simulink model "Parallel_n64"  (R2012b)
settings: Solver=VariableStepDiscrete  StartTime=0.0  StopTime=TotalIterations  RelTol=1e-3
values from neighbouring files (symbols this model uses):
  bp = 12    [ConfigValidate.m]
  bpSNMemory = bp    (= 12)    [ConfigValidate.m]
  IterationsOrdering = 4000    [ConfigValidate.m]
  MaxCoordDistance = (abs(max(wx) - min(wx))+abs(max(wy) - min(wy)))^2    [ConfigValidate.m]
  N_limit = 0.01    [ConfigValidate.m]
  nBits = 9    [ConfigValidate.m]
  nBitsNSmemories = (ceil(log2(TotalIterations)))    [ConfigValidate.m]
  S_limit = 1    [ConfigValidate.m]
  SourceNodes = 2000    [ConfigValidate.m]
  ts = 1    [ConfigValidate.m]
  w1 = rand(1,Neurons)    [ConfigValidate.m]
  w2 = rand(1,Neurons)    [ConfigValidate.m]
  wx = zeros(1,Neurons)    [ConfigValidate.m]
  wy = zeros(1,Neurons)    [ConfigValidate.m]
  x1 = rand(SourceNodes,1)    [ConfigValidate.m]
  x2 = rand(SourceNodes,1)    [ConfigValidate.m]
libraries: xbsIndex_r4 x6367, dspsrcs4 x2, dspstat3 x2
(part 19 of 28)

== system Parallel_n64/WiningNeuronFinder1/LowerDist_n17 ==
  In1 : Inport
  In2 : Inport  Port=2
  In3 : Inport  Port=3
  In4 : Inport  Port=4
  In5 : Inport  Port=5
  In6 : Inport  Port=6
  In7 : Inport  Port=7
  In8 : Inport  Port=8
  In9 : Inport  Port=9
  In10 : Inport  Port=10
  In11 : Inport  Port=11
  In12 : Inport  Port=12
  In13 : Inport  Port=13
  In14 : Inport  Port=14
  In15 : Inport  Port=15
  In16 : Inport  Port=16
  In17 : Inport  Port=17
  In18 : Inport  Port=18
  In19 : Inport  Port=19
  In20 : Inport  Port=20
  In21 : Inport  Port=21
  In22 : Inport  Port=22
  In23 : Inport  Port=23
  In24 : Inport  Port=24
  In25 : Inport  Port=25
  In26 : Inport  Port=26
  In27 : Inport  Port=27
  In28 : Inport  Port=28
  In29 : Inport  Port=29
  In30 : Inport  Port=30
  In31 : Inport  Port=31
  In32 : Inport  Port=32
  In33 : Inport  Port=33
  In34 : Inport  Port=34
  In35 : Inport  Port=35
  In36 : Inport  Port=36
  In37 : Inport  Port=37
  In38 : Inport  Port=38
  In39 : Inport  Port=39
  In40 : Inport  Port=40
  In41 : Inport  Port=41
  In42 : Inport  Port=42
  In43 : Inport  Port=43
  In44 : Inport  Port=44
  In45 : Inport  Port=45
  In46 : Inport  Port=46
  In47 : Inport  Port=47
  In48 : Inport  Port=48
  In49 : Inport  Port=49
  In50 : Inport  Port=50
  In51 : Inport  Port=51
  In52 : Inport  Port=52
  In53 : Inport  Port=53
  In54 : Inport  Port=54
  In55 : Inport  Port=55
  In56 : Inport  Port=56
  In57 : Inport  Port=57
  In58 : Inport  Port=58
  In59 : Inport  Port=59
  In60 : Inport  Port=60
  In61 : Inport  Port=61
  In62 : Inport  Port=62
  In63 : Inport  Port=63
  In64 : Inport  Port=64
  Dist_compare{,1..62} (63 alike) : xbsIndex_r4/Relational  mode=a<=b  en=off  latency=dComparator_CompetitiveProcess  dbl_ovrd=off  block_type=relational
  Logical : xbsIndex_r4/Logical  logical_function=AND  inputs=63  en=off  latency=0  precision=Full  arith_type=Unsigned  n_bits=16  bin_pt=0  align_bp=on  dbl_ovrd=off  block_type=logical
  Out1 : Outport
  wires:
  In24/1 -> Dist_compare19/2
  In23/1 -> Dist_compare18/2
  In17/1 -> Dist_compare15/2
  In16/1 -> Dist_compare14/2
  In14/1 -> Dist_compare12/2
  In12/1 -> Dist_compare10/2
  In11/1 -> Dist_compare9/2
  In10/1 -> Dist_compare8/2
  In8/1 -> Dist_compare6/2
  In22/1 -> Dist_compare17/2
  In13/1 -> Dist_compare11/2
  In9/1 -> Dist_compare7/2
  In20/1 -> Dist_compare24/2
  In21/1 -> Dist_compare16/2
  In19/1 -> Dist_compare23/2
  In18/1 -> Dist_compare22/2
  In25/1 -> Dist_compare20/2
  In15/1 -> Dist_compare13/2
  In2/1 -> Dist_compare/2
  In7/1 -> Dist_compare5/2
  In5/1 -> Dist_compare2/2
  In6/1 -> Dist_compare3/2
  In4/1 -> Dist_compare4/2
  In3/1 -> Dist_compare1/2
  Dist_compare6/1 -> Logical/7
  Dist_compare16/1 -> Logical/20
  Dist_compare14/1 -> Logical/15
  Dist_compare1/1 -> Logical/2
  Dist_compare11/1 -> Logical/12
  Dist_compare/1 -> Logical/1
  Dist_compare24/1 -> Logical/19
  Dist_compare13/1 -> Logical/14
  Dist_compare7/1 -> Logical/8
  Dist_compare4/1 -> Logical/5
  Dist_compare9/1 -> Logical/10
  Dist_compare5/1 -> Logical/6
  Dist_compare18/1 -> Logical/22
  Dist_compare10/1 -> Logical/11
  Dist_compare15/1 -> Logical/16
  Dist_compare23/1 -> Logical/18
  Dist_compare17/1 -> Logical/21
  Dist_compare12/1 -> Logical/13
  Dist_compare20/1 -> Logical/24
  Dist_compare19/1 -> Logical/23
  Logical/1 -> Out1/1
  Dist_compare2/1 -> Logical/3
  Dist_compare22/1 -> Logical/17
  Dist_compare8/1 -> Logical/9
  Dist_compare3/1 -> Logical/4
  In48/1 -> Dist_compare35/2
  In47/1 -> Dist_compare34/2
  In41/1 -> Dist_compare31/2
  In40/1 -> Dist_compare30/2
  In38/1 -> Dist_compare28/2
  In36/1 -> Dist_compare26/2
  In35/1 -> Dist_compare47/2
  In34/1 -> Dist_compare46/2
  In32/1 -> Dist_compare44/2
  In46/1 -> Dist_compare33/2
  In37/1 -> Dist_compare27/2
  In33/1 -> Dist_compare45/2
  In44/1 -> Dist_compare40/2
  In45/1 -> Dist_compare32/2
  In43/1 -> Dist_compare39/2
  In42/1 -> Dist_compare38/2
  In49/1 -> Dist_compare37/2
  In39/1 -> Dist_compare29/2
  In26/1 -> Dist_compare21/2
  In31/1 -> Dist_compare43/2
  In28/1 -> Dist_compare36/2
  In29/1 -> Dist_compare41/2
  In30/1 -> Dist_compare42/2
  In27/1 -> Dist_compare25/2
  In63/1 -> Dist_compare57/2
  In62/1 -> Dist_compare56/2
  In56/1 -> Dist_compare53/2
  In55/1 -> Dist_compare52/2
  In53/1 -> Dist_compare50/2
  In51/1 -> Dist_compare48/2
  In50/1 -> Dist_compare62/2
  In61/1 -> Dist_compare55/2
  In52/1 -> Dist_compare49/2
  In59/1 -> Dist_compare61/2
  In60/1 -> Dist_compare54/2
  In58/1 -> Dist_compare60/2
  In57/1 -> Dist_compare59/2
  In64/1 -> Dist_compare58/2
  In54/1 -> Dist_compare51/2
  In1/1 -> Dist_compare58/1, Dist_compare57/1, Dist_compare56/1, Dist_compare55/1, Dist_compare54/1, Dist_compare61/1, Dist_compare60/1, Dist_compare59/1, Dist_compare53/1, Dist_compare52/1, Dist_compare51/1, Dist_compare50/1, Dist_compare49/1, Dist_compare48/1, Dist_compare62/1, Dist_compare37/1, Dist_compare35/1, Dist_compare34/1, Dist_compare33/1, Dist_compare32/1, Dist_compare40/1, Dist_compare39/1, Dist_compare38/1, Dist_compare31/1, Dist_compare30/1, Dist_compare29/1, Dist_compare28/1, Dist_compare27/1, Dist_compare26/1, Dist_compare47/1, Dist_compare46/1, Dist_compare45/1, Dist_compare44/1, Dist_compare43/1, Dist_compare42/1, Dist_compare41/1, Dist_compare36/1, Dist_compare25/1, Dist_compare21/1, Dist_compare20/1, Dist_compare19/1, Dist_compare18/1, Dist_compare17/1, Dist_compare16/1, Dist_compare24/1, Dist_compare23/1, Dist_compare22/1, Dist_compare15/1, Dist_compare14/1, Dist_compare13/1, Dist_compare12/1, Dist_compare11/1, Dist_compare10/1, Dist_compare9/1, Dist_compare8/1, Dist_compare7/1, Dist_compare6/1, Dist_compare5/1, Dist_compare4/1, Dist_compare3/1, Dist_compare2/1, Dist_compare1/1, Dist_compare/1
  Dist_compare21/1 -> Logical/25
  Dist_compare25/1 -> Logical/26
  Dist_compare36/1 -> Logical/27
  Dist_compare41/1 -> Logical/28
  Dist_compare42/1 -> Logical/29
  Dist_compare43/1 -> Logical/30
  Dist_compare44/1 -> Logical/31
  Dist_compare45/1 -> Logical/32
  Dist_compare46/1 -> Logical/33
  Dist_compare47/1 -> Logical/34
  Dist_compare26/1 -> Logical/35
  Dist_compare27/1 -> Logical/36
  Dist_compare28/1 -> Logical/37
  Dist_compare29/1 -> Logical/38
  Dist_compare30/1 -> Logical/39
  Dist_compare31/1 -> Logical/40
  Dist_compare38/1 -> Logical/41
  Dist_compare39/1 -> Logical/42
  Dist_compare40/1 -> Logical/43
  Dist_compare32/1 -> Logical/44
  Dist_compare33/1 -> Logical/45
  Dist_compare34/1 -> Logical/46
  Dist_compare62/1 -> Logical/49
  Dist_compare35/1 -> Logical/47
  Dist_compare48/1 -> Logical/50
  Dist_compare37/1 -> Logical/48
  Dist_compare50/1 -> Logical/52
  Dist_compare49/1 -> Logical/51
  Dist_compare51/1 -> Logical/53
  Dist_compare52/1 -> Logical/54
  Dist_compare53/1 -> Logical/55
  Dist_compare59/1 -> Logical/56
  Dist_compare60/1 -> Logical/57
  Dist_compare61/1 -> Logical/58
  Dist_compare54/1 -> Logical/59
  Dist_compare56/1 -> Logical/61
  Dist_compare55/1 -> Logical/60
  Dist_compare57/1 -> Logical/62
  Dist_compare58/1 -> Logical/63

== system Parallel_n64/WiningNeuronFinder1/LowerDist_n18 ==
  In1 : Inport
  In2 : Inport  Port=2
  In3 : Inport  Port=3
  In4 : Inport  Port=4
  In5 : Inport  Port=5
  In6 : Inport  Port=6
  In7 : Inport  Port=7
  In8 : Inport  Port=8
  In9 : Inport  Port=9
  In10 : Inport  Port=10
  In11 : Inport  Port=11
  In12 : Inport  Port=12
  In13 : Inport  Port=13
  In14 : Inport  Port=14
  In15 : Inport  Port=15
  In16 : Inport  Port=16
  In17 : Inport  Port=17
  In18 : Inport  Port=18
  In19 : Inport  Port=19
  In20 : Inport  Port=20
  In21 : Inport  Port=21
  In22 : Inport  Port=22
  In23 : Inport  Port=23
  In24 : Inport  Port=24
  In25 : Inport  Port=25
  In26 : Inport  Port=26
  In27 : Inport  Port=27
  In28 : Inport  Port=28
  In29 : Inport  Port=29
  In30 : Inport  Port=30
  In31 : Inport  Port=31
  In32 : Inport  Port=32
  In33 : Inport  Port=33
  In34 : Inport  Port=34
  In35 : Inport  Port=35
  In36 : Inport  Port=36
  In37 : Inport  Port=37
  In38 : Inport  Port=38
  In39 : Inport  Port=39
  In40 : Inport  Port=40
  In41 : Inport  Port=41
  In42 : Inport  Port=42
  In43 : Inport  Port=43
  In44 : Inport  Port=44
  In45 : Inport  Port=45
  In46 : Inport  Port=46
  In47 : Inport  Port=47
  In48 : Inport  Port=48
  In49 : Inport  Port=49
  In50 : Inport  Port=50
  In51 : Inport  Port=51
  In52 : Inport  Port=52
  In53 : Inport  Port=53
  In54 : Inport  Port=54
  In55 : Inport  Port=55
  In56 : Inport  Port=56
  In57 : Inport  Port=57
  In58 : Inport  Port=58
  In59 : Inport  Port=59
  In60 : Inport  Port=60
  In61 : Inport  Port=61
  In62 : Inport  Port=62
  In63 : Inport  Port=63
  In64 : Inport  Port=64
  Dist_compare{,1..62} (63 alike) : xbsIndex_r4/Relational  mode=a<=b  en=off  latency=dComparator_CompetitiveProcess  dbl_ovrd=off  block_type=relational
  Logical : xbsIndex_r4/Logical  logical_function=AND  inputs=63  en=off  latency=0  precision=Full  arith_type=Unsigned  n_bits=16  bin_pt=0  align_bp=on  dbl_ovrd=off  block_type=logical
  Out1 : Outport
  wires:
  In24/1 -> Dist_compare19/2
  In23/1 -> Dist_compare18/2
  In17/1 -> Dist_compare15/2
  In16/1 -> Dist_compare14/2
  In14/1 -> Dist_compare12/2
  In12/1 -> Dist_compare10/2
  In11/1 -> Dist_compare9/2
  In10/1 -> Dist_compare8/2
  In8/1 -> Dist_compare6/2
  In22/1 -> Dist_compare17/2
  In13/1 -> Dist_compare11/2
  In9/1 -> Dist_compare7/2
  In20/1 -> Dist_compare24/2
  In21/1 -> Dist_compare16/2
  In19/1 -> Dist_compare23/2
  In18/1 -> Dist_compare22/2
  In25/1 -> Dist_compare20/2
  In15/1 -> Dist_compare13/2
  In2/1 -> Dist_compare/2
  In7/1 -> Dist_compare5/2
  In5/1 -> Dist_compare2/2
  In6/1 -> Dist_compare3/2
  In4/1 -> Dist_compare4/2
  In3/1 -> Dist_compare1/2
  Dist_compare6/1 -> Logical/7
  Dist_compare16/1 -> Logical/20
  Dist_compare14/1 -> Logical/15
  Dist_compare1/1 -> Logical/2
  Dist_compare11/1 -> Logical/12
  Dist_compare/1 -> Logical/1
  Dist_compare24/1 -> Logical/19
  Dist_compare13/1 -> Logical/14
  Dist_compare7/1 -> Logical/8
  Dist_compare4/1 -> Logical/5
  Dist_compare9/1 -> Logical/10
  Dist_compare5/1 -> Logical/6
  Dist_compare18/1 -> Logical/22
  Dist_compare10/1 -> Logical/11
  Dist_compare15/1 -> Logical/16
  Dist_compare23/1 -> Logical/18
  Dist_compare17/1 -> Logical/21
  Dist_compare12/1 -> Logical/13
  Dist_compare20/1 -> Logical/24
  Dist_compare19/1 -> Logical/23
  Logical/1 -> Out1/1
  Dist_compare2/1 -> Logical/3
  Dist_compare22/1 -> Logical/17
  Dist_compare8/1 -> Logical/9
  Dist_compare3/1 -> Logical/4
  In48/1 -> Dist_compare35/2
  In47/1 -> Dist_compare34/2
  In41/1 -> Dist_compare31/2
  In40/1 -> Dist_compare30/2
  In38/1 -> Dist_compare28/2
  In36/1 -> Dist_compare26/2
  In35/1 -> Dist_compare47/2
  In34/1 -> Dist_compare46/2
  In32/1 -> Dist_compare44/2
  In46/1 -> Dist_compare33/2
  In37/1 -> Dist_compare27/2
  In33/1 -> Dist_compare45/2
  In44/1 -> Dist_compare40/2
  In45/1 -> Dist_compare32/2
  In43/1 -> Dist_compare39/2
  In42/1 -> Dist_compare38/2
  In49/1 -> Dist_compare37/2
  In39/1 -> Dist_compare29/2
  In26/1 -> Dist_compare21/2
  In31/1 -> Dist_compare43/2
  In28/1 -> Dist_compare36/2
  In29/1 -> Dist_compare41/2
  In30/1 -> Dist_compare42/2
  In27/1 -> Dist_compare25/2
  In63/1 -> Dist_compare57/2
  In62/1 -> Dist_compare56/2
  In56/1 -> Dist_compare53/2
  In55/1 -> Dist_compare52/2
  In53/1 -> Dist_compare50/2
  In51/1 -> Dist_compare48/2
  In50/1 -> Dist_compare62/2
  In61/1 -> Dist_compare55/2
  In52/1 -> Dist_compare49/2
  In59/1 -> Dist_compare61/2
  In60/1 -> Dist_compare54/2
  In58/1 -> Dist_compare60/2
  In57/1 -> Dist_compare59/2
  In64/1 -> Dist_compare58/2
  In54/1 -> Dist_compare51/2
  In1/1 -> Dist_compare58/1, Dist_compare57/1, Dist_compare56/1, Dist_compare55/1, Dist_compare54/1, Dist_compare61/1, Dist_compare60/1, Dist_compare59/1, Dist_compare53/1, Dist_compare52/1, Dist_compare51/1, Dist_compare50/1, Dist_compare49/1, Dist_compare48/1, Dist_compare62/1, Dist_compare37/1, Dist_compare35/1, Dist_compare34/1, Dist_compare33/1, Dist_compare32/1, Dist_compare40/1, Dist_compare39/1, Dist_compare38/1, Dist_compare31/1, Dist_compare30/1, Dist_compare29/1, Dist_compare28/1, Dist_compare27/1, Dist_compare26/1, Dist_compare47/1, Dist_compare46/1, Dist_compare45/1, Dist_compare44/1, Dist_compare43/1, Dist_compare42/1, Dist_compare41/1, Dist_compare36/1, Dist_compare25/1, Dist_compare21/1, Dist_compare20/1, Dist_compare19/1, Dist_compare18/1, Dist_compare17/1, Dist_compare16/1, Dist_compare24/1, Dist_compare23/1, Dist_compare22/1, Dist_compare15/1, Dist_compare14/1, Dist_compare13/1, Dist_compare12/1, Dist_compare11/1, Dist_compare10/1, Dist_compare9/1, Dist_compare8/1, Dist_compare7/1, Dist_compare6/1, Dist_compare5/1, Dist_compare4/1, Dist_compare3/1, Dist_compare2/1, Dist_compare1/1, Dist_compare/1
  Dist_compare21/1 -> Logical/25
  Dist_compare25/1 -> Logical/26
  Dist_compare36/1 -> Logical/27
  Dist_compare41/1 -> Logical/28
  Dist_compare42/1 -> Logical/29
  Dist_compare43/1 -> Logical/30
  Dist_compare44/1 -> Logical/31
  Dist_compare45/1 -> Logical/32
  Dist_compare46/1 -> Logical/33
  Dist_compare47/1 -> Logical/34
  Dist_compare26/1 -> Logical/35
  Dist_compare27/1 -> Logical/36
  Dist_compare28/1 -> Logical/37
  Dist_compare29/1 -> Logical/38
  Dist_compare30/1 -> Logical/39
  Dist_compare31/1 -> Logical/40
  Dist_compare38/1 -> Logical/41
  Dist_compare39/1 -> Logical/42
  Dist_compare40/1 -> Logical/43
  Dist_compare32/1 -> Logical/44
  Dist_compare33/1 -> Logical/45
  Dist_compare34/1 -> Logical/46
  Dist_compare62/1 -> Logical/49
  Dist_compare35/1 -> Logical/47
  Dist_compare48/1 -> Logical/50
  Dist_compare37/1 -> Logical/48
  Dist_compare50/1 -> Logical/52
  Dist_compare49/1 -> Logical/51
  Dist_compare51/1 -> Logical/53
  Dist_compare52/1 -> Logical/54
  Dist_compare53/1 -> Logical/55
  Dist_compare59/1 -> Logical/56
  Dist_compare60/1 -> Logical/57
  Dist_compare61/1 -> Logical/58
  Dist_compare54/1 -> Logical/59
  Dist_compare56/1 -> Logical/61
  Dist_compare55/1 -> Logical/60
  Dist_compare57/1 -> Logical/62
  Dist_compare58/1 -> Logical/63

== system Parallel_n64/WiningNeuronFinder1/LowerDist_n19 ==
  In1 : Inport
  In2 : Inport  Port=2
  In3 : Inport  Port=3
  In4 : Inport  Port=4
  In5 : Inport  Port=5
  In6 : Inport  Port=6
  In7 : Inport  Port=7
  In8 : Inport  Port=8
  In9 : Inport  Port=9
  In10 : Inport  Port=10
  In11 : Inport  Port=11
  In12 : Inport  Port=12
  In13 : Inport  Port=13
  In14 : Inport  Port=14
  In15 : Inport  Port=15
  In16 : Inport  Port=16
  In17 : Inport  Port=17
  In18 : Inport  Port=18
  In19 : Inport  Port=19
  In20 : Inport  Port=20
  In21 : Inport  Port=21
  In22 : Inport  Port=22
  In23 : Inport  Port=23
  In24 : Inport  Port=24
  In25 : Inport  Port=25
  In26 : Inport  Port=26
  In27 : Inport  Port=27
  In28 : Inport  Port=28
  In29 : Inport  Port=29
  In30 : Inport  Port=30
  In31 : Inport  Port=31
  In32 : Inport  Port=32
  In33 : Inport  Port=33
  In34 : Inport  Port=34
  In35 : Inport  Port=35
  In36 : Inport  Port=36
  In37 : Inport  Port=37
  In38 : Inport  Port=38
  In39 : Inport  Port=39
  In40 : Inport  Port=40
  In41 : Inport  Port=41
  In42 : Inport  Port=42
  In43 : Inport  Port=43
  In44 : Inport  Port=44
  In45 : Inport  Port=45
  In46 : Inport  Port=46
  In47 : Inport  Port=47
  In48 : Inport  Port=48
  In49 : Inport  Port=49
  In50 : Inport  Port=50
  In51 : Inport  Port=51
  In52 : Inport  Port=52
  In53 : Inport  Port=53
  In54 : Inport  Port=54
  In55 : Inport  Port=55
  In56 : Inport  Port=56
  In57 : Inport  Port=57
  In58 : Inport  Port=58
  In59 : Inport  Port=59
  In60 : Inport  Port=60
  In61 : Inport  Port=61
  In62 : Inport  Port=62
  In63 : Inport  Port=63
  In64 : Inport  Port=64
  Dist_compare{,1..62} (63 alike) : xbsIndex_r4/Relational  mode=a<=b  en=off  latency=dComparator_CompetitiveProcess  dbl_ovrd=off  block_type=relational
  Logical : xbsIndex_r4/Logical  logical_function=AND  inputs=63  en=off  latency=0  precision=Full  arith_type=Unsigned  n_bits=16  bin_pt=0  align_bp=on  dbl_ovrd=off  block_type=logical
  Out1 : Outport
  wires:
  In24/1 -> Dist_compare19/2
  In23/1 -> Dist_compare18/2
  In17/1 -> Dist_compare15/2
  In16/1 -> Dist_compare14/2
  In14/1 -> Dist_compare12/2
  In12/1 -> Dist_compare10/2
  In11/1 -> Dist_compare9/2
  In10/1 -> Dist_compare8/2
  In8/1 -> Dist_compare6/2
  In22/1 -> Dist_compare17/2
  In13/1 -> Dist_compare11/2
  In9/1 -> Dist_compare7/2
  In20/1 -> Dist_compare24/2
  In21/1 -> Dist_compare16/2
  In19/1 -> Dist_compare23/2
  In18/1 -> Dist_compare22/2
  In25/1 -> Dist_compare20/2
  In15/1 -> Dist_compare13/2
  In2/1 -> Dist_compare/2
  In7/1 -> Dist_compare5/2
  In5/1 -> Dist_compare2/2
  In6/1 -> Dist_compare3/2
  In4/1 -> Dist_compare4/2
  In3/1 -> Dist_compare1/2
  Dist_compare6/1 -> Logical/7
  Dist_compare16/1 -> Logical/20
  Dist_compare14/1 -> Logical/15
  Dist_compare1/1 -> Logical/2
  Dist_compare11/1 -> Logical/12
  Dist_compare/1 -> Logical/1
  Dist_compare24/1 -> Logical/19
  Dist_compare13/1 -> Logical/14
  Dist_compare7/1 -> Logical/8
  Dist_compare4/1 -> Logical/5
  Dist_compare9/1 -> Logical/10
  Dist_compare5/1 -> Logical/6
  Dist_compare18/1 -> Logical/22
  Dist_compare10/1 -> Logical/11
  Dist_compare15/1 -> Logical/16
  Dist_compare23/1 -> Logical/18
  Dist_compare17/1 -> Logical/21
  Dist_compare12/1 -> Logical/13
  Dist_compare20/1 -> Logical/24
  Dist_compare19/1 -> Logical/23
  Logical/1 -> Out1/1
  Dist_compare2/1 -> Logical/3
  Dist_compare22/1 -> Logical/17
  Dist_compare8/1 -> Logical/9
  Dist_compare3/1 -> Logical/4
  In48/1 -> Dist_compare35/2
  In47/1 -> Dist_compare34/2
  In41/1 -> Dist_compare31/2
  In40/1 -> Dist_compare30/2
  In38/1 -> Dist_compare28/2
  In36/1 -> Dist_compare26/2
  In35/1 -> Dist_compare47/2
  In34/1 -> Dist_compare46/2
  In32/1 -> Dist_compare44/2
  In46/1 -> Dist_compare33/2
  In37/1 -> Dist_compare27/2
  In33/1 -> Dist_compare45/2
  In44/1 -> Dist_compare40/2
  In45/1 -> Dist_compare32/2
  In43/1 -> Dist_compare39/2
  In42/1 -> Dist_compare38/2
  In49/1 -> Dist_compare37/2
  In39/1 -> Dist_compare29/2
  In26/1 -> Dist_compare21/2
  In31/1 -> Dist_compare43/2
  In28/1 -> Dist_compare36/2
  In29/1 -> Dist_compare41/2
  In30/1 -> Dist_compare42/2
  In27/1 -> Dist_compare25/2
  In63/1 -> Dist_compare57/2
  In62/1 -> Dist_compare56/2
  In56/1 -> Dist_compare53/2
  In55/1 -> Dist_compare52/2
  In53/1 -> Dist_compare50/2
  In51/1 -> Dist_compare48/2
  In50/1 -> Dist_compare62/2
  In61/1 -> Dist_compare55/2
  In52/1 -> Dist_compare49/2
  In59/1 -> Dist_compare61/2
  In60/1 -> Dist_compare54/2
  In58/1 -> Dist_compare60/2
  In57/1 -> Dist_compare59/2
  In64/1 -> Dist_compare58/2
  In54/1 -> Dist_compare51/2
  In1/1 -> Dist_compare58/1, Dist_compare57/1, Dist_compare56/1, Dist_compare55/1, Dist_compare54/1, Dist_compare61/1, Dist_compare60/1, Dist_compare59/1, Dist_compare53/1, Dist_compare52/1, Dist_compare51/1, Dist_compare50/1, Dist_compare49/1, Dist_compare48/1, Dist_compare62/1, Dist_compare37/1, Dist_compare35/1, Dist_compare34/1, Dist_compare33/1, Dist_compare32/1, Dist_compare40/1, Dist_compare39/1, Dist_compare38/1, Dist_compare31/1, Dist_compare30/1, Dist_compare29/1, Dist_compare28/1, Dist_compare27/1, Dist_compare26/1, Dist_compare47/1, Dist_compare46/1, Dist_compare45/1, Dist_compare44/1, Dist_compare43/1, Dist_compare42/1, Dist_compare41/1, Dist_compare36/1, Dist_compare25/1, Dist_compare21/1, Dist_compare20/1, Dist_compare19/1, Dist_compare18/1, Dist_compare17/1, Dist_compare16/1, Dist_compare24/1, Dist_compare23/1, Dist_compare22/1, Dist_compare15/1, Dist_compare14/1, Dist_compare13/1, Dist_compare12/1, Dist_compare11/1, Dist_compare10/1, Dist_compare9/1, Dist_compare8/1, Dist_compare7/1, Dist_compare6/1, Dist_compare5/1, Dist_compare4/1, Dist_compare3/1, Dist_compare2/1, Dist_compare1/1, Dist_compare/1
  Dist_compare21/1 -> Logical/25
  Dist_compare25/1 -> Logical/26
  Dist_compare36/1 -> Logical/27
  Dist_compare41/1 -> Logical/28
  Dist_compare42/1 -> Logical/29
  Dist_compare43/1 -> Logical/30
  Dist_compare44/1 -> Logical/31
  Dist_compare45/1 -> Logical/32
  Dist_compare46/1 -> Logical/33
  Dist_compare47/1 -> Logical/34
  Dist_compare26/1 -> Logical/35
  Dist_compare27/1 -> Logical/36
  Dist_compare28/1 -> Logical/37
  Dist_compare29/1 -> Logical/38
  Dist_compare30/1 -> Logical/39
  Dist_compare31/1 -> Logical/40
  Dist_compare38/1 -> Logical/41
  Dist_compare39/1 -> Logical/42
  Dist_compare40/1 -> Logical/43
  Dist_compare32/1 -> Logical/44
  Dist_compare33/1 -> Logical/45
  Dist_compare34/1 -> Logical/46
  Dist_compare62/1 -> Logical/49
  Dist_compare35/1 -> Logical/47
  Dist_compare48/1 -> Logical/50
  Dist_compare37/1 -> Logical/48
  Dist_compare50/1 -> Logical/52
  Dist_compare49/1 -> Logical/51
  Dist_compare51/1 -> Logical/53
  Dist_compare52/1 -> Logical/54
  Dist_compare53/1 -> Logical/55
  Dist_compare59/1 -> Logical/56
  Dist_compare60/1 -> Logical/57
  Dist_compare61/1 -> Logical/58
  Dist_compare54/1 -> Logical/59
  Dist_compare56/1 -> Logical/61
  Dist_compare55/1 -> Logical/60
  Dist_compare57/1 -> Logical/62
  Dist_compare58/1 -> Logical/63

== system Parallel_n64/WiningNeuronFinder1/LowerDist_n2 ==
  In1 : Inport
  In2 : Inport  Port=2
  In3 : Inport  Port=3
  In4 : Inport  Port=4
  In5 : Inport  Port=5
  In6 : Inport  Port=6
  In7 : Inport  Port=7
  In8 : Inport  Port=8
  In9 : Inport  Port=9
  In10 : Inport  Port=10
  In11 : Inport  Port=11
  In12 : Inport  Port=12
  In13 : Inport  Port=13
  In14 : Inport  Port=14
  In15 : Inport  Port=15
  In16 : Inport  Port=16
  In17 : Inport  Port=17
  In18 : Inport  Port=18
  In19 : Inport  Port=19
  In20 : Inport  Port=20
  In21 : Inport  Port=21
  In22 : Inport  Port=22
  In23 : Inport  Port=23
  In24 : Inport  Port=24
  In25 : Inport  Port=25
  In26 : Inport  Port=26
  In27 : Inport  Port=27
  In28 : Inport  Port=28
  In29 : Inport  Port=29
  In30 : Inport  Port=30
  In31 : Inport  Port=31
  In32 : Inport  Port=32
  In33 : Inport  Port=33
  In34 : Inport  Port=34
  In35 : Inport  Port=35
  In36 : Inport  Port=36
  In37 : Inport  Port=37
  In38 : Inport  Port=38
  In39 : Inport  Port=39
  In40 : Inport  Port=40
  In41 : Inport  Port=41
  In42 : Inport  Port=42
  In43 : Inport  Port=43
  In44 : Inport  Port=44
  In45 : Inport  Port=45
  In46 : Inport  Port=46
  In47 : Inport  Port=47
  In48 : Inport  Port=48
  In49 : Inport  Port=49
  In50 : Inport  Port=50
  In51 : Inport  Port=51
  In52 : Inport  Port=52
  In53 : Inport  Port=53
  In54 : Inport  Port=54
  In55 : Inport  Port=55
  In56 : Inport  Port=56
  In57 : Inport  Port=57
  In58 : Inport  Port=58
  In59 : Inport  Port=59
  In60 : Inport  Port=60
  In61 : Inport  Port=61
  In62 : Inport  Port=62
  In63 : Inport  Port=63
  In64 : Inport  Port=64
  Dist_compare{,1..62} (63 alike) : xbsIndex_r4/Relational  mode=a<=b  en=off  latency=dComparator_CompetitiveProcess  dbl_ovrd=off  block_type=relational
  Logical : xbsIndex_r4/Logical  logical_function=AND  inputs=63  en=off  latency=0  precision=Full  arith_type=Unsigned  n_bits=16  bin_pt=0  align_bp=on  dbl_ovrd=off  block_type=logical
  Out1 : Outport
  wires:
  In24/1 -> Dist_compare19/2
  In23/1 -> Dist_compare18/2
  In17/1 -> Dist_compare15/2
  In16/1 -> Dist_compare14/2
  In14/1 -> Dist_compare12/2
  In12/1 -> Dist_compare10/2
  In11/1 -> Dist_compare9/2
  In10/1 -> Dist_compare8/2
  In8/1 -> Dist_compare6/2
  In22/1 -> Dist_compare17/2
  In13/1 -> Dist_compare11/2
  In9/1 -> Dist_compare7/2
  In20/1 -> Dist_compare24/2
  In21/1 -> Dist_compare16/2
  In19/1 -> Dist_compare23/2
  In18/1 -> Dist_compare22/2
  In25/1 -> Dist_compare20/2
  In15/1 -> Dist_compare13/2
  In2/1 -> Dist_compare/2
  In7/1 -> Dist_compare5/2
  In5/1 -> Dist_compare2/2
  In6/1 -> Dist_compare3/2
  In4/1 -> Dist_compare4/2
  In3/1 -> Dist_compare1/2
  Dist_compare6/1 -> Logical/7
  Dist_compare16/1 -> Logical/20
  Dist_compare14/1 -> Logical/15
  Dist_compare1/1 -> Logical/2
  Dist_compare11/1 -> Logical/12
  Dist_compare/1 -> Logical/1
  Dist_compare24/1 -> Logical/19
  Dist_compare13/1 -> Logical/14
  Dist_compare7/1 -> Logical/8
  Dist_compare4/1 -> Logical/5
  Dist_compare9/1 -> Logical/10
  Dist_compare5/1 -> Logical/6
  Dist_compare18/1 -> Logical/22
  Dist_compare10/1 -> Logical/11
  Dist_compare15/1 -> Logical/16
  Dist_compare23/1 -> Logical/18
  Dist_compare17/1 -> Logical/21
  Dist_compare12/1 -> Logical/13
  Dist_compare20/1 -> Logical/24
  Dist_compare19/1 -> Logical/23
  Logical/1 -> Out1/1
  Dist_compare2/1 -> Logical/3
  Dist_compare22/1 -> Logical/17
  Dist_compare8/1 -> Logical/9
  Dist_compare3/1 -> Logical/4
  In48/1 -> Dist_compare35/2
  In47/1 -> Dist_compare34/2
  In41/1 -> Dist_compare31/2
  In40/1 -> Dist_compare30/2
  In38/1 -> Dist_compare28/2
  In36/1 -> Dist_compare26/2
  In35/1 -> Dist_compare47/2
  In34/1 -> Dist_compare46/2
  In32/1 -> Dist_compare44/2
  In46/1 -> Dist_compare33/2
  In37/1 -> Dist_compare27/2
  In33/1 -> Dist_compare45/2
  In44/1 -> Dist_compare40/2
  In45/1 -> Dist_compare32/2
  In43/1 -> Dist_compare39/2
  In42/1 -> Dist_compare38/2
  In49/1 -> Dist_compare37/2
  In39/1 -> Dist_compare29/2
  In26/1 -> Dist_compare21/2
  In31/1 -> Dist_compare43/2
  In28/1 -> Dist_compare36/2
  In29/1 -> Dist_compare41/2
  In30/1 -> Dist_compare42/2
  In27/1 -> Dist_compare25/2
  In63/1 -> Dist_compare57/2
  In62/1 -> Dist_compare56/2
  In56/1 -> Dist_compare53/2
  In55/1 -> Dist_compare52/2
  In53/1 -> Dist_compare50/2
  In51/1 -> Dist_compare48/2
  In50/1 -> Dist_compare62/2
  In61/1 -> Dist_compare55/2
  In52/1 -> Dist_compare49/2
  In59/1 -> Dist_compare61/2
  In60/1 -> Dist_compare54/2
  In58/1 -> Dist_compare60/2
  In57/1 -> Dist_compare59/2
  In64/1 -> Dist_compare58/2
  In54/1 -> Dist_compare51/2
  In1/1 -> Dist_compare58/1, Dist_compare57/1, Dist_compare56/1, Dist_compare55/1, Dist_compare54/1, Dist_compare61/1, Dist_compare60/1, Dist_compare59/1, Dist_compare53/1, Dist_compare52/1, Dist_compare51/1, Dist_compare50/1, Dist_compare49/1, Dist_compare48/1, Dist_compare62/1, Dist_compare37/1, Dist_compare35/1, Dist_compare34/1, Dist_compare33/1, Dist_compare32/1, Dist_compare40/1, Dist_compare39/1, Dist_compare38/1, Dist_compare31/1, Dist_compare30/1, Dist_compare29/1, Dist_compare28/1, Dist_compare27/1, Dist_compare26/1, Dist_compare47/1, Dist_compare46/1, Dist_compare45/1, Dist_compare44/1, Dist_compare43/1, Dist_compare42/1, Dist_compare41/1, Dist_compare36/1, Dist_compare25/1, Dist_compare21/1, Dist_compare20/1, Dist_compare19/1, Dist_compare18/1, Dist_compare17/1, Dist_compare16/1, Dist_compare24/1, Dist_compare23/1, Dist_compare22/1, Dist_compare15/1, Dist_compare14/1, Dist_compare13/1, Dist_compare12/1, Dist_compare11/1, Dist_compare10/1, Dist_compare9/1, Dist_compare8/1, Dist_compare7/1, Dist_compare6/1, Dist_compare5/1, Dist_compare4/1, Dist_compare3/1, Dist_compare2/1, Dist_compare1/1, Dist_compare/1
  Dist_compare21/1 -> Logical/25
  Dist_compare25/1 -> Logical/26
  Dist_compare36/1 -> Logical/27
  Dist_compare41/1 -> Logical/28
  Dist_compare42/1 -> Logical/29
  Dist_compare43/1 -> Logical/30
  Dist_compare44/1 -> Logical/31
  Dist_compare45/1 -> Logical/32
  Dist_compare46/1 -> Logical/33
  Dist_compare47/1 -> Logical/34
  Dist_compare26/1 -> Logical/35
  Dist_compare27/1 -> Logical/36
  Dist_compare28/1 -> Logical/37
  Dist_compare29/1 -> Logical/38
  Dist_compare30/1 -> Logical/39
  Dist_compare31/1 -> Logical/40
  Dist_compare38/1 -> Logical/41
  Dist_compare39/1 -> Logical/42
  Dist_compare40/1 -> Logical/43
  Dist_compare32/1 -> Logical/44
  Dist_compare33/1 -> Logical/45
  Dist_compare34/1 -> Logical/46
  Dist_compare62/1 -> Logical/49
  Dist_compare35/1 -> Logical/47
  Dist_compare48/1 -> Logical/50
  Dist_compare37/1 -> Logical/48
  Dist_compare50/1 -> Logical/52
  Dist_compare49/1 -> Logical/51
  Dist_compare51/1 -> Logical/53
  Dist_compare52/1 -> Logical/54
  Dist_compare53/1 -> Logical/55
  Dist_compare59/1 -> Logical/56
  Dist_compare60/1 -> Logical/57
  Dist_compare61/1 -> Logical/58
  Dist_compare54/1 -> Logical/59
  Dist_compare56/1 -> Logical/61
  Dist_compare55/1 -> Logical/60
  Dist_compare57/1 -> Logical/62
  Dist_compare58/1 -> Logical/63

== system Parallel_n64/WiningNeuronFinder1/LowerDist_n20 ==
  In1 : Inport
  In2 : Inport  Port=2
  In3 : Inport  Port=3
  In4 : Inport  Port=4
  In5 : Inport  Port=5
  In6 : Inport  Port=6
  In7 : Inport  Port=7
  In8 : Inport  Port=8
  In9 : Inport  Port=9
  In10 : Inport  Port=10
  In11 : Inport  Port=11
  In12 : Inport  Port=12
  In13 : Inport  Port=13
  In14 : Inport  Port=14
  In15 : Inport  Port=15
  In16 : Inport  Port=16
  In17 : Inport  Port=17
  In18 : Inport  Port=18
  In19 : Inport  Port=19
  In20 : Inport  Port=20
  In21 : Inport  Port=21
  In22 : Inport  Port=22
  In23 : Inport  Port=23
  In24 : Inport  Port=24
  In25 : Inport  Port=25
  In26 : Inport  Port=26
  In27 : Inport  Port=27
  In28 : Inport  Port=28
  In29 : Inport  Port=29
  In30 : Inport  Port=30
  In31 : Inport  Port=31
  In32 : Inport  Port=32
  In33 : Inport  Port=33
  In34 : Inport  Port=34
  In35 : Inport  Port=35
  In36 : Inport  Port=36
  In37 : Inport  Port=37
  In38 : Inport  Port=38
  In39 : Inport  Port=39
  In40 : Inport  Port=40
  In41 : Inport  Port=41
  In42 : Inport  Port=42
  In43 : Inport  Port=43
  In44 : Inport  Port=44
  In45 : Inport  Port=45
  In46 : Inport  Port=46
  In47 : Inport  Port=47
  In48 : Inport  Port=48
  In49 : Inport  Port=49
  In50 : Inport  Port=50
  In51 : Inport  Port=51
  In52 : Inport  Port=52
  In53 : Inport  Port=53
  In54 : Inport  Port=54
  In55 : Inport  Port=55
  In56 : Inport  Port=56
  In57 : Inport  Port=57
  In58 : Inport  Port=58
  In59 : Inport  Port=59
  In60 : Inport  Port=60
  In61 : Inport  Port=61
  In62 : Inport  Port=62
  In63 : Inport  Port=63
  In64 : Inport  Port=64
  Dist_compare{,1..62} (63 alike) : xbsIndex_r4/Relational  mode=a<=b  en=off  latency=dComparator_CompetitiveProcess  dbl_ovrd=off  block_type=relational
  Logical : xbsIndex_r4/Logical  logical_function=AND  inputs=63  en=off  latency=0  precision=Full  arith_type=Unsigned  n_bits=16  bin_pt=0  align_bp=on  dbl_ovrd=off  block_type=logical
  Out1 : Outport
  wires:
  In24/1 -> Dist_compare19/2
  In23/1 -> Dist_compare18/2
  In17/1 -> Dist_compare15/2
  In16/1 -> Dist_compare14/2
  In14/1 -> Dist_compare12/2
  In12/1 -> Dist_compare10/2
  In11/1 -> Dist_compare9/2
  In10/1 -> Dist_compare8/2
  In8/1 -> Dist_compare6/2
  In22/1 -> Dist_compare17/2
  In13/1 -> Dist_compare11/2
  In9/1 -> Dist_compare7/2
  In20/1 -> Dist_compare24/2
  In21/1 -> Dist_compare16/2
  In19/1 -> Dist_compare23/2
  In18/1 -> Dist_compare22/2
  In25/1 -> Dist_compare20/2
  In15/1 -> Dist_compare13/2
  In2/1 -> Dist_compare/2
  In7/1 -> Dist_compare5/2
  In5/1 -> Dist_compare2/2
  In6/1 -> Dist_compare3/2
  In4/1 -> Dist_compare4/2
  In3/1 -> Dist_compare1/2
  Dist_compare6/1 -> Logical/7
  Dist_compare16/1 -> Logical/20
  Dist_compare14/1 -> Logical/15
  Dist_compare1/1 -> Logical/2
  Dist_compare11/1 -> Logical/12
  Dist_compare/1 -> Logical/1
  Dist_compare24/1 -> Logical/19
  Dist_compare13/1 -> Logical/14
  Dist_compare7/1 -> Logical/8
  Dist_compare4/1 -> Logical/5
  Dist_compare9/1 -> Logical/10
  Dist_compare5/1 -> Logical/6
  Dist_compare18/1 -> Logical/22
  Dist_compare10/1 -> Logical/11
  Dist_compare15/1 -> Logical/16
  Dist_compare23/1 -> Logical/18
  Dist_compare17/1 -> Logical/21
  Dist_compare12/1 -> Logical/13
  Dist_compare20/1 -> Logical/24
  Dist_compare19/1 -> Logical/23
  Logical/1 -> Out1/1
  Dist_compare2/1 -> Logical/3
  Dist_compare22/1 -> Logical/17
  Dist_compare8/1 -> Logical/9
  Dist_compare3/1 -> Logical/4
  In48/1 -> Dist_compare35/2
  In47/1 -> Dist_compare34/2
  In41/1 -> Dist_compare31/2
  In40/1 -> Dist_compare30/2
  In38/1 -> Dist_compare28/2
  In36/1 -> Dist_compare26/2
  In35/1 -> Dist_compare47/2
  In34/1 -> Dist_compare46/2
  In32/1 -> Dist_compare44/2
  In46/1 -> Dist_compare33/2
  In37/1 -> Dist_compare27/2
  In33/1 -> Dist_compare45/2
  In44/1 -> Dist_compare40/2
  In45/1 -> Dist_compare32/2
  In43/1 -> Dist_compare39/2
  In42/1 -> Dist_compare38/2
  In49/1 -> Dist_compare37/2
  In39/1 -> Dist_compare29/2
  In26/1 -> Dist_compare21/2
  In31/1 -> Dist_compare43/2
  In28/1 -> Dist_compare36/2
  In29/1 -> Dist_compare41/2
  In30/1 -> Dist_compare42/2
  In27/1 -> Dist_compare25/2
  In63/1 -> Dist_compare57/2
  In62/1 -> Dist_compare56/2
  In56/1 -> Dist_compare53/2
  In55/1 -> Dist_compare52/2
  In53/1 -> Dist_compare50/2
  In51/1 -> Dist_compare48/2
  In50/1 -> Dist_compare62/2
  In61/1 -> Dist_compare55/2
  In52/1 -> Dist_compare49/2
  In59/1 -> Dist_compare61/2
  In60/1 -> Dist_compare54/2
  In58/1 -> Dist_compare60/2
  In57/1 -> Dist_compare59/2
  In64/1 -> Dist_compare58/2
  In54/1 -> Dist_compare51/2
  In1/1 -> Dist_compare58/1, Dist_compare57/1, Dist_compare56/1, Dist_compare55/1, Dist_compare54/1, Dist_compare61/1, Dist_compare60/1, Dist_compare59/1, Dist_compare53/1, Dist_compare52/1, Dist_compare51/1, Dist_compare50/1, Dist_compare49/1, Dist_compare48/1, Dist_compare62/1, Dist_compare37/1, Dist_compare35/1, Dist_compare34/1, Dist_compare33/1, Dist_compare32/1, Dist_compare40/1, Dist_compare39/1, Dist_compare38/1, Dist_compare31/1, Dist_compare30/1, Dist_compare29/1, Dist_compare28/1, Dist_compare27/1, Dist_compare26/1, Dist_compare47/1, Dist_compare46/1, Dist_compare45/1, Dist_compare44/1, Dist_compare43/1, Dist_compare42/1, Dist_compare41/1, Dist_compare36/1, Dist_compare25/1, Dist_compare21/1, Dist_compare20/1, Dist_compare19/1, Dist_compare18/1, Dist_compare17/1, Dist_compare16/1, Dist_compare24/1, Dist_compare23/1, Dist_compare22/1, Dist_compare15/1, Dist_compare14/1, Dist_compare13/1, Dist_compare12/1, Dist_compare11/1, Dist_compare10/1, Dist_compare9/1, Dist_compare8/1, Dist_compare7/1, Dist_compare6/1, Dist_compare5/1, Dist_compare4/1, Dist_compare3/1, Dist_compare2/1, Dist_compare1/1, Dist_compare/1
  Dist_compare21/1 -> Logical/25
  Dist_compare25/1 -> Logical/26
  Dist_compare36/1 -> Logical/27
  Dist_compare41/1 -> Logical/28
  Dist_compare42/1 -> Logical/29
  Dist_compare43/1 -> Logical/30
  Dist_compare44/1 -> Logical/31
  Dist_compare45/1 -> Logical/32
  Dist_compare46/1 -> Logical/33
  Dist_compare47/1 -> Logical/34
  Dist_compare26/1 -> Logical/35
  Dist_compare27/1 -> Logical/36
  Dist_compare28/1 -> Logical/37
  Dist_compare29/1 -> Logical/38
  Dist_compare30/1 -> Logical/39
  Dist_compare31/1 -> Logical/40
  Dist_compare38/1 -> Logical/41
  Dist_compare39/1 -> Logical/42
  Dist_compare40/1 -> Logical/43
  Dist_compare32/1 -> Logical/44
  Dist_compare33/1 -> Logical/45
  Dist_compare34/1 -> Logical/46
  Dist_compare62/1 -> Logical/49
  Dist_compare35/1 -> Logical/47
  Dist_compare48/1 -> Logical/50
  Dist_compare37/1 -> Logical/48
  Dist_compare50/1 -> Logical/52
  Dist_compare49/1 -> Logical/51
  Dist_compare51/1 -> Logical/53
  Dist_compare52/1 -> Logical/54
  Dist_compare53/1 -> Logical/55
  Dist_compare59/1 -> Logical/56
  Dist_compare60/1 -> Logical/57
  Dist_compare61/1 -> Logical/58
  Dist_compare54/1 -> Logical/59
  Dist_compare56/1 -> Logical/61
  Dist_compare55/1 -> Logical/60
  Dist_compare57/1 -> Logical/62
  Dist_compare58/1 -> Logical/63

== system Parallel_n64/WiningNeuronFinder1/LowerDist_n21 ==
  In1 : Inport
  In2 : Inport  Port=2
  In3 : Inport  Port=3
  In4 : Inport  Port=4
  In5 : Inport  Port=5
  In6 : Inport  Port=6
  In7 : Inport  Port=7
  In8 : Inport  Port=8
  In9 : Inport  Port=9
  In10 : Inport  Port=10
  In11 : Inport  Port=11
  In12 : Inport  Port=12
  In13 : Inport  Port=13
  In14 : Inport  Port=14
  In15 : Inport  Port=15
  In16 : Inport  Port=16
  In17 : Inport  Port=17
  In18 : Inport  Port=18
  In19 : Inport  Port=19
  In20 : Inport  Port=20
  In21 : Inport  Port=21
  In22 : Inport  Port=22
  In23 : Inport  Port=23
  In24 : Inport  Port=24
  In25 : Inport  Port=25
  In26 : Inport  Port=26
  In27 : Inport  Port=27
  In28 : Inport  Port=28
  In29 : Inport  Port=29
  In30 : Inport  Port=30
  In31 : Inport  Port=31
  In32 : Inport  Port=32
  In33 : Inport  Port=33
  In34 : Inport  Port=34
  In35 : Inport  Port=35
  In36 : Inport  Port=36
  In37 : Inport  Port=37
  In38 : Inport  Port=38
  In39 : Inport  Port=39
  In40 : Inport  Port=40
  In41 : Inport  Port=41
  In42 : Inport  Port=42
  In43 : Inport  Port=43
  In44 : Inport  Port=44
  In45 : Inport  Port=45
  In46 : Inport  Port=46
  In47 : Inport  Port=47
  In48 : Inport  Port=48
  In49 : Inport  Port=49
  In50 : Inport  Port=50
  In51 : Inport  Port=51
  In52 : Inport  Port=52
  In53 : Inport  Port=53
  In54 : Inport  Port=54
  In55 : Inport  Port=55
  In56 : Inport  Port=56
  In57 : Inport  Port=57
  In58 : Inport  Port=58
  In59 : Inport  Port=59
  In60 : Inport  Port=60
  In61 : Inport  Port=61
  In62 : Inport  Port=62
  In63 : Inport  Port=63
  In64 : Inport  Port=64
  Dist_compare{,1..62} (63 alike) : xbsIndex_r4/Relational  mode=a<=b  en=off  latency=dComparator_CompetitiveProcess  dbl_ovrd=off  block_type=relational
  Logical : xbsIndex_r4/Logical  logical_function=AND  inputs=63  en=off  latency=0  precision=Full  arith_type=Unsigned  n_bits=16  bin_pt=0  align_bp=on  dbl_ovrd=off  block_type=logical
  Out1 : Outport
  wires:
  In24/1 -> Dist_compare19/2
  In23/1 -> Dist_compare18/2
  In17/1 -> Dist_compare15/2
  In16/1 -> Dist_compare14/2
  In14/1 -> Dist_compare12/2
  In12/1 -> Dist_compare10/2
  In11/1 -> Dist_compare9/2
  In10/1 -> Dist_compare8/2
  In8/1 -> Dist_compare6/2
  In22/1 -> Dist_compare17/2
  In13/1 -> Dist_compare11/2
  In9/1 -> Dist_compare7/2
  In20/1 -> Dist_compare24/2
  In21/1 -> Dist_compare16/2
  In19/1 -> Dist_compare23/2
  In18/1 -> Dist_compare22/2
  In25/1 -> Dist_compare20/2
  In15/1 -> Dist_compare13/2
  In2/1 -> Dist_compare/2
  In7/1 -> Dist_compare5/2
  In5/1 -> Dist_compare2/2
  In6/1 -> Dist_compare3/2
  In4/1 -> Dist_compare4/2
  In3/1 -> Dist_compare1/2
  Dist_compare6/1 -> Logical/7
  Dist_compare16/1 -> Logical/20
  Dist_compare14/1 -> Logical/15
  Dist_compare1/1 -> Logical/2
  Dist_compare11/1 -> Logical/12
  Dist_compare/1 -> Logical/1
  Dist_compare24/1 -> Logical/19
  Dist_compare13/1 -> Logical/14
  Dist_compare7/1 -> Logical/8
  Dist_compare4/1 -> Logical/5
  Dist_compare9/1 -> Logical/10
  Dist_compare5/1 -> Logical/6
  Dist_compare18/1 -> Logical/22
  Dist_compare10/1 -> Logical/11
  Dist_compare15/1 -> Logical/16
  Dist_compare23/1 -> Logical/18
  Dist_compare17/1 -> Logical/21
  Dist_compare12/1 -> Logical/13
  Dist_compare20/1 -> Logical/24
  Dist_compare19/1 -> Logical/23
  Logical/1 -> Out1/1
  Dist_compare2/1 -> Logical/3
  Dist_compare22/1 -> Logical/17
  Dist_compare8/1 -> Logical/9
  Dist_compare3/1 -> Logical/4
  In48/1 -> Dist_compare35/2
  In47/1 -> Dist_compare34/2
  In41/1 -> Dist_compare31/2
  In40/1 -> Dist_compare30/2
  In38/1 -> Dist_compare28/2
  In36/1 -> Dist_compare26/2
  In35/1 -> Dist_compare47/2
  In34/1 -> Dist_compare46/2
  In32/1 -> Dist_compare44/2
  In46/1 -> Dist_compare33/2
  In37/1 -> Dist_compare27/2
  In33/1 -> Dist_compare45/2
  In44/1 -> Dist_compare40/2
  In45/1 -> Dist_compare32/2
  In43/1 -> Dist_compare39/2
  In42/1 -> Dist_compare38/2
  In49/1 -> Dist_compare37/2
  In39/1 -> Dist_compare29/2
  In26/1 -> Dist_compare21/2
  In31/1 -> Dist_compare43/2
  In28/1 -> Dist_compare36/2
  In29/1 -> Dist_compare41/2
  In30/1 -> Dist_compare42/2
  In27/1 -> Dist_compare25/2
  In63/1 -> Dist_compare57/2
  In62/1 -> Dist_compare56/2
  In56/1 -> Dist_compare53/2
  In55/1 -> Dist_compare52/2
  In53/1 -> Dist_compare50/2
  In51/1 -> Dist_compare48/2
  In50/1 -> Dist_compare62/2
  In61/1 -> Dist_compare55/2
  In52/1 -> Dist_compare49/2
  In59/1 -> Dist_compare61/2
  In60/1 -> Dist_compare54/2
  In58/1 -> Dist_compare60/2
  In57/1 -> Dist_compare59/2
  In64/1 -> Dist_compare58/2
  In54/1 -> Dist_compare51/2
  In1/1 -> Dist_compare58/1, Dist_compare57/1, Dist_compare56/1, Dist_compare55/1, Dist_compare54/1, Dist_compare61/1, Dist_compare60/1, Dist_compare59/1, Dist_compare53/1, Dist_compare52/1, Dist_compare51/1, Dist_compare50/1, Dist_compare49/1, Dist_compare48/1, Dist_compare62/1, Dist_compare37/1, Dist_compare35/1, Dist_compare34/1, Dist_compare33/1, Dist_compare32/1, Dist_compare40/1, Dist_compare39/1, Dist_compare38/1, Dist_compare31/1, Dist_compare30/1, Dist_compare29/1, Dist_compare28/1, Dist_compare27/1, Dist_compare26/1, Dist_compare47/1, Dist_compare46/1, Dist_compare45/1, Dist_compare44/1, Dist_compare43/1, Dist_compare42/1, Dist_compare41/1, Dist_compare36/1, Dist_compare25/1, Dist_compare21/1, Dist_compare20/1, Dist_compare19/1, Dist_compare18/1, Dist_compare17/1, Dist_compare16/1, Dist_compare24/1, Dist_compare23/1, Dist_compare22/1, Dist_compare15/1, Dist_compare14/1, Dist_compare13/1, Dist_compare12/1, Dist_compare11/1, Dist_compare10/1, Dist_compare9/1, Dist_compare8/1, Dist_compare7/1, Dist_compare6/1, Dist_compare5/1, Dist_compare4/1, Dist_compare3/1, Dist_compare2/1, Dist_compare1/1, Dist_compare/1
  Dist_compare21/1 -> Logical/25
  Dist_compare25/1 -> Logical/26
  Dist_compare36/1 -> Logical/27
  Dist_compare41/1 -> Logical/28
  Dist_compare42/1 -> Logical/29
  Dist_compare43/1 -> Logical/30
  Dist_compare44/1 -> Logical/31
  Dist_compare45/1 -> Logical/32
  Dist_compare46/1 -> Logical/33
  Dist_compare47/1 -> Logical/34
  Dist_compare26/1 -> Logical/35
  Dist_compare27/1 -> Logical/36
  Dist_compare28/1 -> Logical/37
  Dist_compare29/1 -> Logical/38
  Dist_compare30/1 -> Logical/39
  Dist_compare31/1 -> Logical/40
  Dist_compare38/1 -> Logical/41
  Dist_compare39/1 -> Logical/42
  Dist_compare40/1 -> Logical/43
  Dist_compare32/1 -> Logical/44
  Dist_compare33/1 -> Logical/45
  Dist_compare34/1 -> Logical/46
  Dist_compare62/1 -> Logical/49
  Dist_compare35/1 -> Logical/47
  Dist_compare48/1 -> Logical/50
  Dist_compare37/1 -> Logical/48
  Dist_compare50/1 -> Logical/52
  Dist_compare49/1 -> Logical/51
  Dist_compare51/1 -> Logical/53
  Dist_compare52/1 -> Logical/54
  Dist_compare53/1 -> Logical/55
  Dist_compare59/1 -> Logical/56
  Dist_compare60/1 -> Logical/57
  Dist_compare61/1 -> Logical/58
  Dist_compare54/1 -> Logical/59
  Dist_compare56/1 -> Logical/61
  Dist_compare55/1 -> Logical/60
  Dist_compare57/1 -> Logical/62
  Dist_compare58/1 -> Logical/63
